simulink model "SC_Lab1_Variant3"  (R2025b)
settings: Solver=ode45  StartTime=0.0  StopTime=1  RelTol=1e-3
settings Model: Creator=m  LastModifiedBy=m
settings DataIOCC: SaveFormat=StructureWithTime

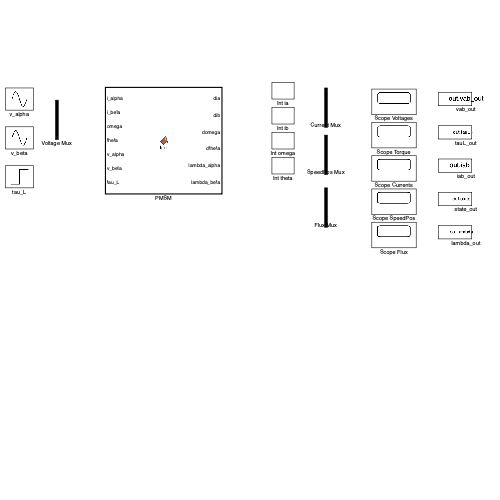
[thumbnail: Simulink's stored preview of the top-level diagram]
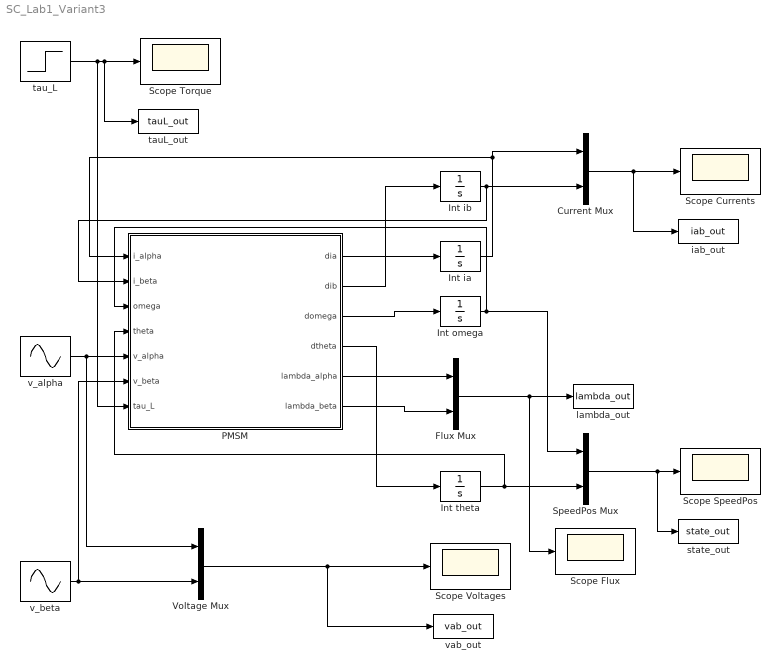
== system SC_Lab1_Variant3 ==
  Current Mux : Mux  Inputs=2
  Flux Mux : Mux  Inputs=2
  Int ia : Integrator
  Int ib : Integrator
  Int omega : Integrator
  Int theta : Integrator
  PMSM : MATLAB Function  TreatAsAtomicUnit=on
  Scope Currents : Scope
  Scope Flux : Scope
  Scope SpeedPos : Scope
  Scope Torque : Scope
  Scope Voltages : Scope
  SpeedPos Mux : Mux  Inputs=2
  Voltage Mux : Mux  Inputs=2
  iab_out : ToWorkspace  VariableName=iab_out  SaveFormat=Structure With Time  SampleTime=-1
  lambda_out : ToWorkspace  VariableName=lambda_out  SaveFormat=Structure With Time  SampleTime=-1
  state_out : ToWorkspace  VariableName=state_out  SaveFormat=Structure With Time  SampleTime=-1
  tauL_out : ToWorkspace  VariableName=tauL_out  SaveFormat=Structure With Time  SampleTime=-1
  tau_L : Step  Time=0.5  After=0.35  SampleTime=0
  v_alpha : Sin  Amplitude=52  Frequency=26  Phase=pi/2  SampleTime=0
  v_beta : Sin  Amplitude=52  Frequency=26  SampleTime=0
  vab_out : ToWorkspace  VariableName=vab_out  SaveFormat=Structure With Time  SampleTime=-1
  wires:
  SpeedPos Mux/1 -> state_out/1, Scope SpeedPos/1
  Current Mux/1 -> iab_out/1, Scope Currents/1
  Int theta/1 -> SpeedPos Mux/2, PMSM/4(theta)
  Flux Mux/1 -> lambda_out/1, Scope Flux/1
  Int omega/1 -> SpeedPos Mux/1, PMSM/3(omega)
  PMSM/5(lambda_alpha) -> Flux Mux/1
  v_beta/1 -> PMSM/6(v_beta), Voltage Mux/2
  PMSM/4(dtheta) -> Int theta/1
  Int ib/1 -> Current Mux/2, PMSM/2(i_beta)
  PMSM/2(dib) -> Int ib/1
  PMSM/3(domega) -> Int omega/1
  PMSM/1(dia) -> Int ia/1
  tau_L/1 -> tauL_out/1, Scope Torque/1, PMSM/7(tau_L)
  Voltage Mux/1 -> vab_out/1, Scope Voltages/1
  v_alpha/1 -> PMSM/5(v_alpha), Voltage Mux/1
  Int ia/1 -> Current Mux/1, PMSM/1(i_alpha)
  PMSM/6(lambda_beta) -> Flux Mux/2

== matlab function SC_Lab1_Variant3/PMSM ==
  data: i_alpha input; dia output; i_beta input; omega input; theta input; v_alpha input; v_beta input; tau_L input; dib output; domega output; dtheta output; lambda_alpha output; lambda_beta output
function [dia, dib, domega, dtheta, lambda_alpha, lambda_beta] = fcn(i_alpha, i_beta, omega, theta, v_alpha, v_beta, tau_L)
                                                                                                                          L = 0.033;                                                                                                                 
                                                                                                                          R = 5.3;                                                                                                                   
                                                                                                                          Jm = 0.0006;                                                                                                               
                                                                                                                          np = 5;                                                                                                                    
                                                                                                                          lambda_m = 0.16;                                                                                                           
                                                                                                                          B = 0;                                                                                                                     
                                                                                                                          theta_e = np * theta;                                                                                                      
                                                                                                                          c = cos(theta_e);                                                                                                          
                                                                                                                          s = sin(theta_e);                                                                                                          
                                                                                                                          dia = (-R*i_alpha + v_alpha + lambda_m*np*omega*s) / L;                                                                    
                                                                                                                          dib = (-R*i_beta + v_beta - lambda_m*np*omega*c) / L;                                                                      
                                                                                                                          tau_e = np * lambda_m * (-i_alpha*s + i_beta*c);                                                                           
                                                                                                                          domega = (-B*omega + tau_e - tau_L) / Jm;                                                                                  
                                                                                                                          dtheta = omega;                                                                                                            
                                                                                                                          lambda_alpha = L*i_alpha + lambda_m*c;                                                                                     
                                                                                                                          lambda_beta = L*i_beta + lambda_m*s;
